simulink model "duty_cycle"  (R2019a)
settings: Solver=VariableStepAuto  StartTime=0.0  StopTime=0.1/60  RelTol=1e-3
libraries: powerlib_meascontrol x1
settings Model: Creator=Ram Baskar  LastModifiedBy=Ram Baskar

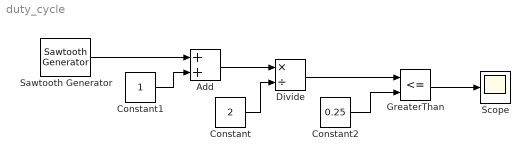
== system duty_cycle ==
  Add : Sum
  Constant : Constant  Value=2
  Constant1 : Constant
  Constant2 : Constant  Value=0.25
  Divide : Product  Inputs=*/
  GreaterThan : RelationalOperator  Operator=<=  OutDataTypeStr=boolean  RndMeth=Simplest
  Sawtooth Generator : powerlib_meascontrol/Pulse & Signal Generators/Sawtooth Generator  Freq=1e3  Phase=0  Ts=0
      settings: SourceProductName=Simscape Electrical
  Scope : Scope
  wires:
  Sawtooth Generator/1 -> Add/1
  Constant1/1 -> Add/2
  Add/1 -> Divide/1
  Constant/1 -> Divide/2
  Constant2/1 -> GreaterThan/2
  Divide/1 -> GreaterThan/1
  GreaterThan/1 -> Scope/1
